simulink model "sample_speed_velocity"  (R2020b)
settings: Solver=FixedStepAuto  StartTime=0.0  StopTime=2  FixedStep=0.00001  RelTol=1e-3
undefined symbols (not defined in the file): B, CoulombAndViscousFriction, J_eq, K_tau, n_1, r_3, switch_on
settings Model: PacingRate=0.001000  Creator=Bens PC  LastModifiedBy=Bens PC

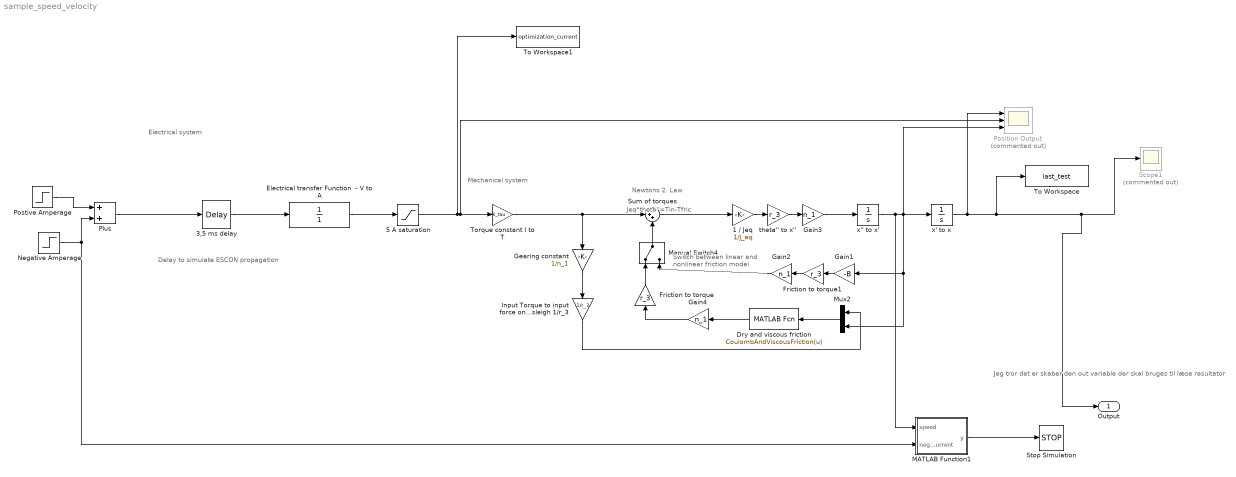
== system sample_speed_velocity ==
  note: Jeg tror det er skaber den out variable der skal bruges til læse resultator
  note: Switch between linear
      | and nonlinear friction model
  note: Newtons 2. Law
  note: Delay to simulate ESCON propagation
  note: Electrical system
  note: Jeq*theta''=Tin-Tfric
  note: Mechanical system
  1 / Jeq : Gain  Gain=1/J_eq
  3,5 ms delay : TransportDelay  DelayTime=0.0035
  5 A saturation : Saturate  UpperLimit=5  LowerLimit=-5
  Dry and viscous friction : MATLABFcn  MATLABFcn=CoulombAndViscousFriction(u)  OutputDimensions=1
  Electrical transfer Function  - V to A : TransferFcn  Denominator=[1]
  Friction to torque : Gain  Gain=r_3
  Friction to torque1 : Gain  Gain=r_3
  Gain1 : Gain  Gain=-B
  Gain2 : Gain  Gain=n_1
  Gain3 : Gain  Gain=n_1
  Gain4 : Gain  Gain=n_1
  Gearing constant : Gain  Gain=1/n_1
  Input Torque to input force on sleigh 1/r_3 : Gain  Gain=1/r_3
  MATLAB Function1 : MATLAB Function  TreatAsAtomicUnit=on
  Manual Switch4 : ManualSwitch
  Mux2 : Mux  Inputs=2
  Negative Amperage : Step  Time=switch_on  After=-10  SampleTime=0
  Plus : Sum
  Position Output : Scope  Commented=on  NumInputPorts=3
  Postive Amperage : Step  Time=0  After=5  SampleTime=0
  Scope1 : Scope  Commented=on
  Stop Simulation : Stop
  Sum of torques : Sum  Inputs=|++
  To Workspace : ToWorkspace  VariableName=last_test  SaveFormat=Timeseries  SampleTime=-1
  To Workspace1 : ToWorkspace  VariableName=optimization_current  SaveFormat=Timeseries  SampleTime=-1
  "Torque constant I to T " : Gain  Gain=K_tau
  theta'' to x'' : Gain  Gain=r_3
  x' to x : Integrator
  x'' to x' : Integrator
  Output : Outport
  wires:
  Gain3/1 -> x'' to x'/1
  "Torque constant I to T "/1 -> Sum of torques/1, Gearing constant/1
  Gain2/1 -> Manual Switch4/2
  Input Torque to input force on sleigh 1/r_3/1 -> Mux2/1
  Electrical transfer Function  - V to A/1 -> 5 A saturation/1
  x' to x/1 -> To Workspace/1, Scope1/1, Output/1, Position Output/1
  1 / Jeq/1 -> theta'' to x''/1
  Gain1/1 -> Friction to torque1/1
  Friction to torque/1 -> Manual Switch4/1
  Manual Switch4/1 -> Sum of torques/2
  Gearing constant/1 -> Input Torque to input force on sleigh 1/r_3/1
  Gain4/1 -> Friction to torque/1
  3,5 ms delay/1 -> Electrical transfer Function  - V to A/1
  Dry and viscous friction/1 -> Gain4/1
  theta'' to x''/1 -> Gain3/1
  x'' to x'/1 -> MATLAB Function1/1(speed), Position Output/3, Gain1/1, Mux2/2, x' to x/1
  Friction to torque1/1 -> Gain2/1
  5 A saturation/1 -> To Workspace1/1, Position Output/2, "Torque constant I to T "/1
  Mux2/1 -> Dry and viscous friction/1
  Sum of torques/1 -> 1 / Jeq/1
  Plus/1 -> 3,5 ms delay/1
  MATLAB Function1/1(y) -> Stop Simulation/1
  Postive Amperage/1 -> Plus/1
  Negative Amperage/1 -> MATLAB Function1/2(negative_current), Plus/2

== matlab function sample_speed_velocity/MATLAB Function1 ==
  data: y output; speed input; negative_current input
function y = fcn(speed, negative_current)



if (abs(speed) < 0.01) && (negative_current ~= 0)
    y = 1;
else
    y = 0;
end
